simulink model "progetto2_mi_dist_kalm2"  (Simulink 7.9)
settings: Solver=ode45  StartTime=0.0  StopTime=30  RelTol=1e-3
values from neighbouring files (symbols this model uses):
  A = [0 0 0 0 0 0 0 -9.80999999984 0 0 0 0 ... (144 elements, 12x12)]    [A.mat]    (also in QuadLqrAstat105.m = loadA.A; Tenzo1_05.m = [ 0 0 0 1 0 0 0 0 0 0 0 0)
  Aoss = A-V*C    [QuadLqrAstat105.m]
  Boss = [B-V*D V]    [QuadLqrAstat105.m]
  C = [0 0 0 0 0 0 1 0 0 0 0 0 ... (144 elements, 12x12)]    [C.mat]    (also in QuadLqrAstat105.m = loadC.C)
  Coss = eye(size(A))    [QuadLqrAstat105.m]
  Doss = zeros(size(Boss))    [QuadLqrAstat105.m]
  omega = 4    [QuadLqrAstat105.m]    (also in Tenzo1_05.m)
undefined symbols (not defined in the file or in its folder): AMI, BMI, Bmod, CMI, DMI, Dmod, F1, F2
settings Model: Creator=danilo  LastModifiedBy=userk
settings DebuggingCC: FcnCallInpInsideContextMsg=Use local settings
settings GRTTargetCC: CombineOutputUpdateFcns=off  GRTInterface=on

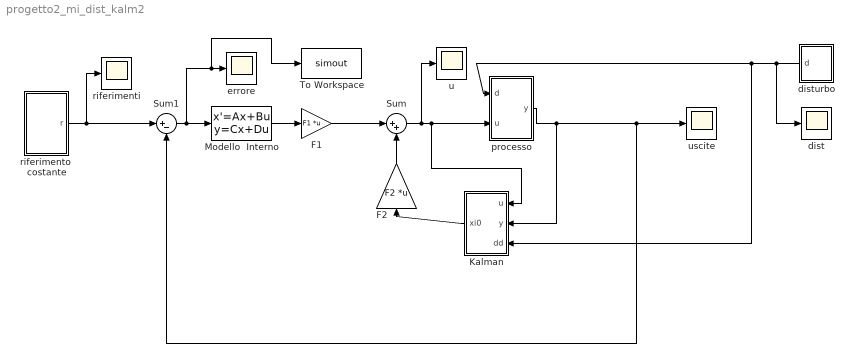
== system progetto2_mi_dist_kalm2 ==
  F1 : Gain  Gain=F1  Multiplication=Matrix(K*u) (u vector)
  F2 : Gain  Gain=F2  Multiplication=Matrix(K*u) (u vector)
  Kalman : Subsystem
  Modello  Interno : StateSpace  A=AMI  B=BMI  C=CMI  D=DMI
  Sum : Sum  Inputs=|++
  Sum1 : Sum  Inputs=|+-
  To Workspace : ToWorkspace  VariableName=simout  SampleTime=-1  SaveFormat=Structure
  dist : Scope
      settings: SaveName=ScopeData5
  disturbo : Subsystem
  errore : Scope
      settings: SaveName=ScopeData2
  processo : Subsystem
  riferimenti : Scope
  riferimento  costante : Subsystem
  u : Scope
      settings: SaveName=ScopeData3
  uscite : Scope
      settings: YMin=0.75  YMax=4.25
  wires:
  riferimento  costante/1(r) -> Sum1/1, riferimenti/1
  processo/1(y) -> uscite/1, Sum1/2, Kalman/2(y)
  Kalman/1(xi0) -> F2/1
  Modello  Interno/1 -> F1/1
  F2/1 -> Sum/2
  F1/1 -> Sum/1
  Sum/1 -> Kalman/1(u), processo/2(u), u/1
  Sum1/1 -> Modello  Interno/1, errore/1, To Workspace/1
  disturbo/1(d) -> dist/1, processo/1(d), Kalman/3(dd)

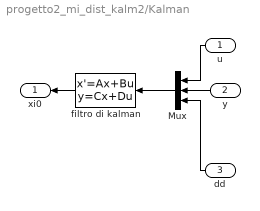
== system progetto2_mi_dist_kalm2/Kalman ==
  u : Inport
  y : Inport  Port=2
  dd : Inport  Port=3
  Mux : Mux  Inputs=[2 2 1]
  filtro di kalman : StateSpace  A=Aoss  B=Boss  C=Coss  D=Doss
  xi0 : Outport
  wires:
  Mux/1 -> filtro di kalman/1
  u/1 -> Mux/1
  filtro di kalman/1 -> xi0/1
  y/1 -> Mux/2
  dd/1 -> Mux/3

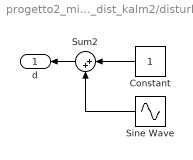
== system progetto2_mi_dist_kalm2/disturbo ==
  Constant : Constant
  Sine Wave : Sin  Frequency=omega  SampleTime=0
  Sum2 : Sum  Inputs=|++
  d : Outport
  wires:
  Sine Wave/1 -> Sum2/2
  Constant/1 -> Sum2/1
  Sum2/1 -> d/1

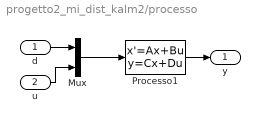
== system progetto2_mi_dist_kalm2/processo ==
  d : Inport
  u : Inport  Port=2
  Mux : Mux  Inputs=[1 2]
  Processo1 : StateSpace  A=A  B=Bmod  C=C  D=Dmod
  y : Outport
  wires:
  Mux/1 -> Processo1/1
  d/1 -> Mux/1
  Processo1/1 -> y/1
  u/1 -> Mux/2

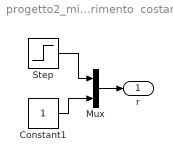
== system progetto2_mi_dist_kalm2/riferimento  costante ==
  Constant1 : Constant
  Mux : Mux  Inputs=[1 1]
  Step : Step  Time=3  After=4  SampleTime=0
  r : Outport
  wires:
  Mux/1 -> r/1
  Step/1 -> Mux/1
  Constant1/1 -> Mux/2
